simulink model "Number_7"  (R2023b)
settings: Solver=VariableStepAuto  StartTime=0.0  StopTime=20  RelTol=1e-3
values from neighbouring files (symbols this model uses):
  G_den7 = [1 2 3 4 5 1]    [Number_7_8.m]
  G_num7 = [6 5 4 3 2]    [Number_7_8.m]
settings Model: Creator=Mariven Amurao  LastModifiedBy=Mariven Amurao

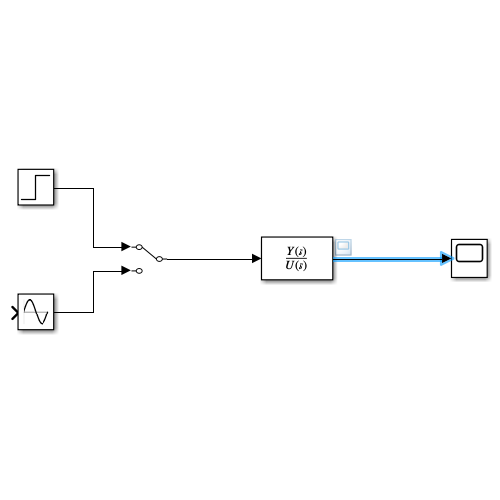
[thumbnail: Simulink's stored preview of the top-level diagram]
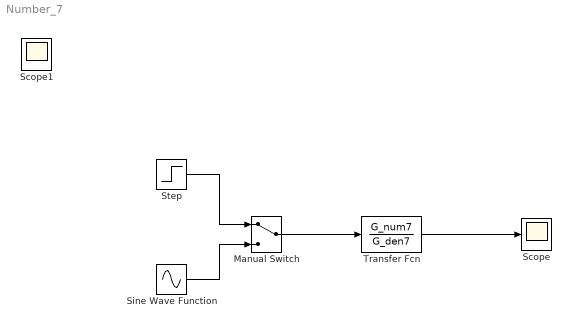
== system Number_7 ==
  Manual Switch : ManualSwitch
  Scope : Scope
  Sine Wave Function : Sin  TimeSource=Use external signal  SampleTime=0
  Step : Step  SampleTime=0
  Transfer Fcn : TransferFcn  Numerator=G_num7  Denominator=G_den7
  Scope1 : Scope
  wires:
  Manual Switch/1 -> Transfer Fcn/1
  Sine Wave Function/1 -> Manual Switch/2
  Step/1 -> Manual Switch/1
  Transfer Fcn/1 -> Scope/1
